simulink model "CubliSenseToolSim"  (R2017b)
settings: Solver=FixedStepAuto  StartTime=0.0  StopTime=5  FixedStep=0.0025  RelTol=1e-3  EnableMultiTasking=on
values from neighbouring files (symbols this model uses):
  B_f = 6.08e-3    (= 0.00608)    [CubliSenseTool.m]
  g = 9.82    [CubliSenseTool.m]
  init_theta = 0.1286    [CubliSenseTool.m]
  J_f = 2.8e-3    (= 0.0028)    [CubliSenseTool.m]
  J_w = 0.601e-3    (= 0.000601)    [CubliSenseTool.m]
  l_f = 0.08498    [CubliSenseTool.m]
  l_w = 0.093    [CubliSenseTool.m]
  m_f = 0.77-m_w    (= 0.548)    [CubliSenseTool.m]
  m_w = 0.222    [CubliSenseTool.m]
settings Model: Creator=vniel  LastModifiedBy=niels
settings DataIOCC: SaveFormat=Array  Refine=25
settings OptimizationCC: LifeSpan=inf
settings DebuggingCC: AllowSymbolicDim=off  SFUnexpectedBacktrackingDiag=warning  SFNoUnconditionalDefaultTransitionDiag=warning  SFExecutionAtInitializationDiag=none
settings HardwareCC: ProdBitPerPointer=32  ProdBitPerSizeT=32  ProdBitPerPtrDiffT=32  ProdLargestAtomicFloat=None  ProdIntDivRoundTo=Undefined  ProdEndianess=Unspecified  ProdWordSize=32  ProdHWDeviceType=32-bit Generic
settings ModelReferenceCC: PropagateSignalLabelsOutOfModel=off
settings CodeAppCC: StateflowObjectComments=on
settings GRTTargetCC: TargetLangStandard=C89/C90 (ANSI)  GeneratePreprocessorConditionals=Disable all
settings ConfigComp: CovMetricSettings=dw  CovHtmlReporting=on  CovSaveCumulativeToWorkspaceVar=on  CovSaveSingleToWorkspaceVar=on  CovExternalEMLEnable=off

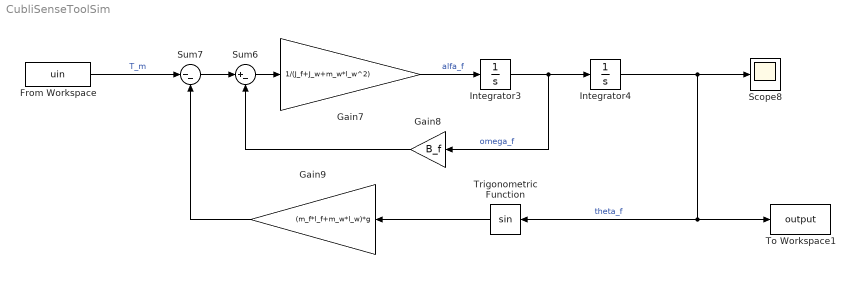
== system CubliSenseToolSim ==
  From Workspace : FromWorkspace  VariableName=uin
  Gain7 : Gain  Gain=1/(J_f+J_w+m_w*l_w^2)
  Gain8 : Gain  Gain=B_f
  Gain9 : Gain  Gain=(m_f*l_f+m_w*l_w)*g
  Integrator3 : Integrator
  Integrator4 : Integrator  InitialCondition=init_theta
  Scope8 : Scope
  Sum6 : Sum  Inputs=|+-
  Sum7 : Sum  Inputs=|--
  To Workspace1 : ToWorkspace  VariableName=output  SampleTime=0.0025
      settings: MaxDataPoints=2000
  Trigonometric Function : Trigonometry
  wires:
  Gain7/1 -> Integrator3/1  "alfa_f"
  Integrator3/1 -> Gain8/1, Integrator4/1  "omega_f"
  Sum6/1 -> Gain7/1
  Sum7/1 -> Sum6/1
  Gain8/1 -> Sum6/2
  Gain9/1 -> Sum7/2
  Integrator4/1 -> To Workspace1/1, Trigonometric Function/1, Scope8/1  "theta_f"
  Trigonometric Function/1 -> Gain9/1
  From Workspace/1 -> Sum7/1  "T_m"
